simulink model "CG_Xilinxmodel"  (R2014a)
settings: Solver=ode45  StartTime=0.0  StopTime=0.12  RelTol=1e-3
undefined symbols (not defined in the file or in its folder): Down, Up
libraries: xbsIndex_r4 x102, powerlib x21
settings Model: Creator=Kiruba  LastModifiedBy=Acer
settings DebuggingCC: UnderspecifiedInitializationDetection=Classic

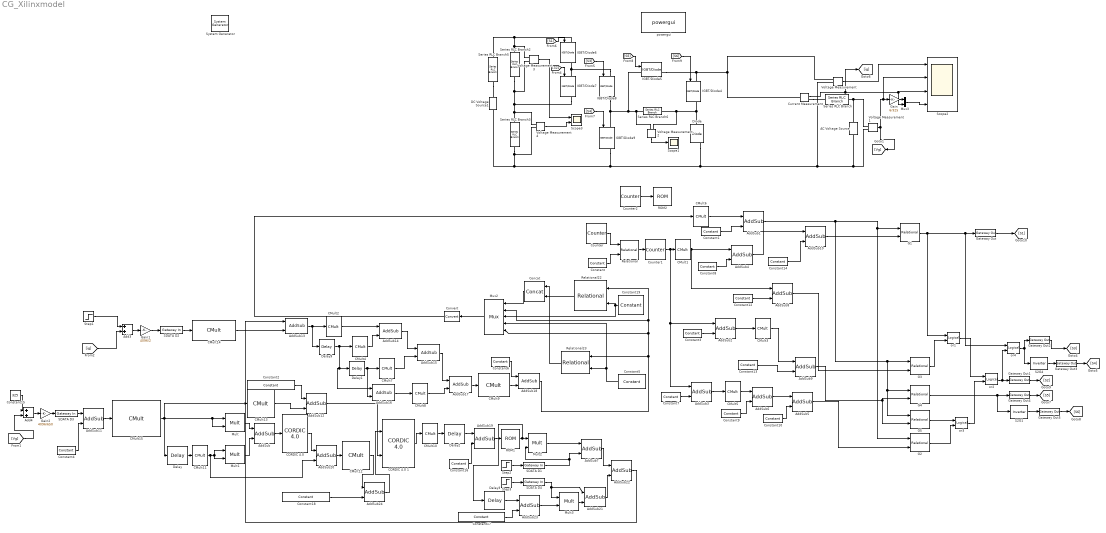
== system CG_Xilinxmodel ==
  " System Generator" : xbsIndex_r4/ System Generator  Tag=genX  xilinxfamily=spartan6  part=xc6slx45  speed=-3  package=csg324  synthesis_tool=XST  clock_wrapper=Clock Enables  directory=./netlist  proj_type=Project Navigator  Synth_file=XST Defaults  Impl_file=ISE Defaults  testbench=off  simulink_period=10e-9  sysclk_period=10  dcm_input_clock_period=10  incr_netlist=off  trim_vbits=Everywhere in SubSystem  dbl_ovrd=According to Block Masks  core_generation=According to Block Masks  run_coregen=off  deprecated_control=off  eval_field=0  block_type=sysgen
  AC Voltage Source : powerlib/Electrical Sources/AC Voltage Source  Amplitude=325  Phase=0  Frequency=50  SampleTime=0  Measurements=None
  Add3 : Sum
  Add4 : Sum
  AddSub : xbsIndex_r4/AddSub  mode=Addition  use_carryin=off  use_carryout=off  en=off  latency=0  precision=User Defined  arith_type=Unsigned  n_bits=18  bin_pt=0  quantization=Truncate  overflow=Wrap  dbl_ovrd=off  use_behavioral_HDL=off  hw_selection=Fabric  pipelined=off  block_type=addsub
  AddSub1 : xbsIndex_r4/AddSub  mode=Addition  use_carryin=off  use_carryout=off  en=off  latency=0  precision=Full  arith_type="Signed  (2's comp)"  n_bits=60  bin_pt=30  quantization=Truncate  overflow=Wrap  dbl_ovrd=off  use_behavioral_HDL=off  hw_selection=Fabric  pipelined=off  block_type=addsub
  AddSub10 : xbsIndex_r4/AddSub  mode=Addition  use_carryin=off  use_carryout=off  en=off  latency=0  precision=Full  arith_type="Signed  (2's comp)"  n_bits=60  bin_pt=30  quantization=Truncate  overflow=Wrap  dbl_ovrd=off  use_behavioral_HDL=off  hw_selection=Fabric  pipelined=off  block_type=addsub
  AddSub11 : xbsIndex_r4/AddSub  mode=Subtraction  use_carryin=off  use_carryout=off  en=off  latency=0  precision=Full  arith_type=Unsigned  n_bits=16  bin_pt=14  quantization=Truncate  overflow=Wrap  dbl_ovrd=off  use_behavioral_HDL=off  hw_selection=Fabric  pipelined=off  block_type=addsub
  AddSub12 : xbsIndex_r4/AddSub  mode=Addition  use_carryin=off  use_carryout=off  en=off  latency=0  precision=User Defined  arith_type="Signed  (2's comp)"  n_bits=32  bin_pt=30  quantization=Truncate  overflow=Wrap  dbl_ovrd=off  use_behavioral_HDL=off  hw_selection=Fabric  pipelined=off  block_type=addsub
  AddSub13 : xbsIndex_r4/AddSub  mode=Subtraction  use_carryin=off  use_carryout=off  en=off  latency=0  precision=Full  arith_type=Unsigned  n_bits=16  bin_pt=14  quantization=Truncate  overflow=Wrap  dbl_ovrd=off  use_behavioral_HDL=off  hw_selection=Fabric  pipelined=off  block_type=addsub
  AddSub{7,14..15,17..18,21..22} (7 alike) : xbsIndex_r4/AddSub  mode=Addition  use_carryin=off  use_carryout=off  en=off  latency=0  precision=Full  arith_type=Unsigned  n_bits=16  bin_pt=14  quantization=Truncate  overflow=Wrap  dbl_ovrd=off  use_behavioral_HDL=off  hw_selection=Fabric  pipelined=off  block_type=addsub
  AddSub16 : xbsIndex_r4/AddSub  mode=Subtraction  use_carryin=off  use_carryout=off  en=off  latency=1  precision=Full  arith_type=Unsigned  n_bits=16  bin_pt=14  quantization=Truncate  overflow=Wrap  dbl_ovrd=off  use_behavioral_HDL=off  hw_selection=Fabric  pipelined=off  block_type=addsub
  AddSub19 : xbsIndex_r4/AddSub  mode=Addition  use_carryin=off  use_carryout=off  en=off  latency=0  precision=User Defined  arith_type=Unsigned  n_bits=14  bin_pt=0  quantization=Truncate  overflow=Wrap  dbl_ovrd=off  use_behavioral_HDL=off  hw_selection=Fabric  pipelined=off  block_type=addsub
  AddSub2 : xbsIndex_r4/AddSub  mode=Subtraction  use_carryin=off  use_carryout=off  en=off  latency=0  precision=Full  arith_type=Unsigned  n_bits=13  bin_pt=0  quantization=Truncate  overflow=Wrap  dbl_ovrd=off  use_behavioral_HDL=off  hw_selection=Fabric  pipelined=off  block_type=addsub
  AddSub20 : xbsIndex_r4/AddSub  mode=Subtraction  use_carryin=off  use_carryout=off  en=off  latency=0  precision=Full  arith_type="Signed  (2's comp)"  n_bits=9  bin_pt=7  quantization=Truncate  overflow=Wrap  dbl_ovrd=off  use_behavioral_HDL=off  hw_selection=Fabric  pipelined=off  block_type=addsub
  AddSub23 : xbsIndex_r4/AddSub  mode=Addition  use_carryin=off  use_carryout=off  en=off  latency=0  precision=User Defined  arith_type="Signed  (2's comp)"  n_bits=32  bin_pt=30  quantization=Truncate  overflow=Wrap  dbl_ovrd=off  use_behavioral_HDL=off  hw_selection=Fabric  pipelined=off  block_type=addsub
  AddSub24 : xbsIndex_r4/AddSub  mode=Addition  use_carryin=off  use_carryout=off  en=off  latency=0  precision=User Defined  arith_type="Signed  (2's comp)"  n_bits=32  bin_pt=30  quantization=Truncate  overflow=Wrap  dbl_ovrd=off  use_behavioral_HDL=off  hw_selection=Fabric  pipelined=off  block_type=addsub
  AddSub3 : xbsIndex_r4/AddSub  mode=Subtraction  use_carryin=off  use_carryout=off  en=off  latency=0  precision=Full  arith_type=Unsigned  n_bits=13  bin_pt=0  quantization=Truncate  overflow=Wrap  dbl_ovrd=off  use_behavioral_HDL=off  hw_selection=Fabric  pipelined=off  block_type=addsub
  AddSub{4..5,8..9} (4 alike) : xbsIndex_r4/AddSub  mode=Addition  use_carryin=off  use_carryout=off  en=off  latency=0  precision=Full  arith_type=Unsigned  n_bits=13  bin_pt=0  quantization=Truncate  overflow=Wrap  dbl_ovrd=off  use_behavioral_HDL=off  hw_selection=Fabric  pipelined=off  block_type=addsub
  AddSub6 : xbsIndex_r4/AddSub  mode=Subtraction  use_carryin=off  use_carryout=off  en=off  latency=0  precision=Full  arith_type=Unsigned  n_bits=13  bin_pt=0  quantization=Truncate  overflow=Wrap  dbl_ovrd=off  use_behavioral_HDL=off  hw_selection=Fabric  pipelined=off  block_type=addsub
  CMult1 : xbsIndex_r4/CMult  const=0.5  gui_display_data_type=Fixed-point  const_n_bits=16  const_bin_pt=4  float_type=Single  exp_bits=8  fraction_bits=24  en=off  latency=0  precision=Full  arith_type="Signed  (2's comp)"  n_bits=16  bin_pt=14  quantization=Truncate  overflow=Wrap  dbl_ovrd=off  use_behavioral_HDL=off  mem_type=Distributed RAM  pipeline=off  block_type=cmult
      settings: block_version=12.1
  CMult10 : xbsIndex_r4/CMult  const=-250  gui_display_data_type=Fixed-point  const_n_bits=10  const_bin_pt=0  float_type=Single  exp_bits=8  fraction_bits=24  en=off  latency=0  precision=Full  arith_type="Signed  (2's comp)"  n_bits=16  bin_pt=14  quantization=Truncate  overflow=Wrap  dbl_ovrd=off  use_behavioral_HDL=off  mem_type=Distributed RAM  pipeline=off  block_type=cmult
      settings: block_version=12.1
  CMult11 : xbsIndex_r4/CMult  const=-1  gui_display_data_type=Fixed-point  const_n_bits=9  const_bin_pt=0  float_type=Single  exp_bits=8  fraction_bits=24  en=off  latency=0  precision=Full  arith_type="Signed  (2's comp)"  n_bits=16  bin_pt=14  quantization=Truncate  overflow=Wrap  dbl_ovrd=off  use_behavioral_HDL=off  mem_type=Distributed RAM  pipeline=off  block_type=cmult
      settings: block_version=12.1
  CMult12 : xbsIndex_r4/CMult  const=1/650  gui_display_data_type=Fixed-point  const_n_bits=32  const_bin_pt=30  float_type=Single  exp_bits=8  fraction_bits=24  en=off  latency=0  precision=User Defined  arith_type="Signed  (2's comp)"  n_bits=32  bin_pt=30  quantization=Truncate  overflow=Wrap  dbl_ovrd=off  use_behavioral_HDL=off  mem_type=Distributed RAM  pipeline=off  block_type=cmult
  CMult13 : xbsIndex_r4/CMult  const=1/650  gui_display_data_type=Fixed-point  const_n_bits=32  const_bin_pt=30  float_type=Single  exp_bits=8  fraction_bits=24  en=off  latency=0  precision=User Defined  arith_type="Signed  (2's comp)"  n_bits=9  bin_pt=7  quantization=Truncate  overflow=Wrap  dbl_ovrd=off  use_behavioral_HDL=off  mem_type=Distributed RAM  pipeline=off  block_type=cmult
  CMult14 : xbsIndex_r4/CMult  const=2/4096  gui_display_data_type=Fixed-point  const_n_bits=20  const_bin_pt=18  float_type=Single  exp_bits=8  fraction_bits=24  en=off  latency=0  precision=Full  arith_type="Signed  (2's comp)"  n_bits=16  bin_pt=14  quantization=Truncate  overflow=Wrap  dbl_ovrd=off  use_behavioral_HDL=off  mem_type=Distributed RAM  pipeline=off  block_type=cmult
      settings: block_version=12.1
  CMult15 : xbsIndex_r4/CMult  const=650/4101  gui_display_data_type=Fixed-point  const_n_bits=20  const_bin_pt=18  float_type=Single  exp_bits=8  fraction_bits=24  en=off  latency=0  precision=Full  arith_type="Signed  (2's comp)"  n_bits=16  bin_pt=14  quantization=Truncate  overflow=Wrap  dbl_ovrd=off  use_behavioral_HDL=off  mem_type=Distributed RAM  pipeline=off  block_type=cmult
      settings: block_version=12.1
  CMult2 : xbsIndex_r4/CMult  const=250.5  gui_display_data_type=Fixed-point  const_n_bits=10  const_bin_pt=2  float_type=Single  exp_bits=8  fraction_bits=24  en=off  latency=0  precision=Full  arith_type="Signed  (2's comp)"  n_bits=16  bin_pt=14  quantization=Truncate  overflow=Wrap  dbl_ovrd=off  use_behavioral_HDL=off  mem_type=Distributed RAM  pipeline=off  block_type=cmult
      settings: block_version=12.1
  CMult3 : xbsIndex_r4/CMult  const=0.5  gui_display_data_type=Fixed-point  const_n_bits=16  const_bin_pt=4  float_type=Single  exp_bits=8  fraction_bits=24  en=off  latency=0  precision=Full  arith_type="Signed  (2's comp)"  n_bits=16  bin_pt=14  quantization=Truncate  overflow=Wrap  dbl_ovrd=off  use_behavioral_HDL=off  mem_type=Distributed RAM  pipeline=off  block_type=cmult
      settings: block_version=12.1
  CMult4 : xbsIndex_r4/CMult  const=180.2  gui_display_data_type=Fixed-point  const_n_bits=10  const_bin_pt=2  float_type=Single  exp_bits=8  fraction_bits=24  en=off  latency=0  precision=Full  arith_type="Signed  (2's comp)"  n_bits=16  bin_pt=14  quantization=Truncate  overflow=Wrap  dbl_ovrd=off  use_behavioral_HDL=off  mem_type=Distributed RAM  pipeline=off  block_type=cmult
      settings: block_version=12.1
  CMult5 : xbsIndex_r4/CMult  const=0.5  gui_display_data_type=Fixed-point  const_n_bits=16  const_bin_pt=4  float_type=Single  exp_bits=8  fraction_bits=24  en=off  latency=0  precision=Full  arith_type="Signed  (2's comp)"  n_bits=16  bin_pt=14  quantization=Truncate  overflow=Wrap  dbl_ovrd=off  use_behavioral_HDL=off  mem_type=Distributed RAM  pipeline=off  block_type=cmult
      settings: block_version=12.1
  CMult6 : xbsIndex_r4/CMult  const=1250  gui_display_data_type=Fixed-point  const_n_bits=16  const_bin_pt=4  float_type=Single  exp_bits=8  fraction_bits=24  en=off  latency=0  precision=Full  arith_type="Signed  (2's comp)"  n_bits=16  bin_pt=14  quantization=Truncate  overflow=Wrap  dbl_ovrd=off  use_behavioral_HDL=off  mem_type=Distributed RAM  pipeline=off  block_type=cmult
      settings: block_version=12.1
  CMult7 : xbsIndex_r4/CMult  const=15.5  gui_display_data_type=Fixed-point  const_n_bits=10  const_bin_pt=2  float_type=Single  exp_bits=8  fraction_bits=24  en=off  latency=0  precision=Full  arith_type="Signed  (2's comp)"  n_bits=16  bin_pt=14  quantization=Truncate  overflow=Wrap  dbl_ovrd=off  use_behavioral_HDL=off  mem_type=Distributed RAM  pipeline=off  block_type=cmult
      settings: block_version=12.1
  CMult8 : xbsIndex_r4/CMult  const=2  gui_display_data_type=Fixed-point  const_n_bits=10  const_bin_pt=2  float_type=Single  exp_bits=8  fraction_bits=24  en=off  latency=0  precision=Full  arith_type="Signed  (2's comp)"  n_bits=16  bin_pt=14  quantization=Truncate  overflow=Wrap  dbl_ovrd=off  use_behavioral_HDL=off  mem_type=Distributed RAM  pipeline=off  block_type=cmult
      settings: block_version=12.1
  CMult9 : xbsIndex_r4/CMult  const=(1/400)  gui_display_data_type=Fixed-point  const_n_bits=14  const_bin_pt=12  float_type=Single  exp_bits=8  fraction_bits=24  en=off  latency=0  precision=Full  arith_type="Signed  (2's comp)"  n_bits=16  bin_pt=14  quantization=Truncate  overflow=Wrap  dbl_ovrd=off  use_behavioral_HDL=off  mem_type=Distributed RAM  pipeline=off  block_type=cmult
      settings: block_version=12.1
  "CORDIC 4.0 " : xbsIndex_r4/CORDIC 4.0   functional_selection=Square_Root  architectural_configuration=Parallel  pipelining_mode=Maximum  data_format=UnsignedInteger  phase_format=Radians  output_width=10  round_mode=Truncate  iterations=0  precision=0  coarse_rotation=off  compensation_scaling=No_Scale_Compensation  ce=off  sclr=off  nd=off  rdy=off  x_out=on  y_out=off  phase_output=off  register_inputs=true  register_outputs=true  ipcore_usecache=true  ipcore_useipmodelcache=true  ipcore_verbose=false  wrapper_available=true  ip_name=CORDIC  ip_version=4.0  dsptool_ready=true  port_translation_map={ 'ce' => 'en', 'sclr' => 'rst' }  structural_sim=false  block_type=cordic_v4_0
  CORDIC 4.0 1 : xbsIndex_r4/CORDIC 4.0   functional_selection=Arc_Tan  architectural_configuration=Parallel  pipelining_mode=No_Pipelining  data_format=SignedFraction  phase_format=Radians  output_width=40  round_mode=Truncate  iterations=0  precision=0  coarse_rotation=on  compensation_scaling=No_Scale_Compensation  ce=off  sclr=off  nd=off  rdy=off  x_out=off  y_out=off  phase_output=on  register_inputs=true  register_outputs=true  ipcore_usecache=true  ipcore_useipmodelcache=true  ipcore_verbose=false  wrapper_available=true  ip_name=CORDIC  ip_version=4.0  dsptool_ready=true  port_translation_map={ 'ce' => 'en', 'sclr' => 'rst' }  structural_sim=false  block_type=cordic_v4_0
  Concat : xbsIndex_r4/Concat  num_inputs=2  dbl_ovrd=off  block_type=concat
  Constant : xbsIndex_r4/Constant  const=1250  gui_display_data_type=Fixed-point  arith_type=Unsigned  n_bits=16  bin_pt=0  preci_type=Single  exp_width=8  frac_width=24  explicit_period=off  period=1  equ=P=C  opselect=C  inp2=PCIN>>17  opr=+  inp1=P  carry=CIN  dbl_ovrd=off  block_type=constant
  Constant1 : xbsIndex_r4/Constant  const=0  gui_display_data_type=Fixed-point  arith_type=Unsigned  n_bits=30  bin_pt=4  preci_type=Single  exp_width=8  frac_width=24  explicit_period=off  period=1  equ=P=C  opselect=C  inp2=PCIN>>17  opr=+  inp1=P  carry=CIN  dbl_ovrd=off  block_type=constant
      settings: block_version=12.1
  Constant{3,7,10,12..13} (5 alike) : xbsIndex_r4/Constant  const=1250  gui_display_data_type=Fixed-point  arith_type=Unsigned  n_bits=13  bin_pt=2  preci_type=Single  exp_width=8  frac_width=24  explicit_period=off  period=1  equ=P=C  opselect=C  inp2=PCIN>>17  opr=+  inp1=P  carry=CIN  dbl_ovrd=off  block_type=constant
      settings: block_version=12.1
  Constant14 : xbsIndex_r4/Constant  const=1250  gui_display_data_type=Fixed-point  arith_type=Unsigned  n_bits=30  bin_pt=4  preci_type=Single  exp_width=8  frac_width=24  explicit_period=off  period=1  equ=P=C  opselect=C  inp2=PCIN>>17  opr=+  inp1=P  carry=CIN  dbl_ovrd=off  block_type=constant
      settings: block_version=12.1
  Constant15 : Constant  Value=325
  Constant16 : xbsIndex_r4/Constant  const=393  gui_display_data_type=Fixed-point  arith_type=Unsigned  n_bits=10  bin_pt=0  preci_type=Single  exp_width=8  frac_width=24  explicit_period=off  period=1  equ=P=C  opselect=C  inp2=PCIN>>17  opr=+  inp1=P  carry=CIN  dbl_ovrd=off  block_type=constant
  Constant17 : xbsIndex_r4/Constant  const=0.06  gui_display_data_type=Fixed-point  arith_type=Signed (2's comp)  n_bits=32  bin_pt=30  preci_type=Single  exp_width=8  frac_width=24  explicit_period=off  period=1  equ=P=C  opselect=C  inp2=PCIN>>17  opr=+  inp1=P  carry=CIN  dbl_ovrd=off  block_type=constant
  Constant18 : xbsIndex_r4/Constant  const=0.00108  gui_display_data_type=Fixed-point  arith_type=Signed (2's comp)  n_bits=32  bin_pt=30  preci_type=Single  exp_width=8  frac_width=24  explicit_period=off  period=1  equ=P=C  opselect=C  inp2=PCIN>>17  opr=+  inp1=P  carry=CIN  dbl_ovrd=off  block_type=constant
  Constant19 : xbsIndex_r4/Constant  const=2  gui_display_data_type=Fixed-point  arith_type=Signed (2's comp)  n_bits=15  bin_pt=10  preci_type=Single  exp_width=8  frac_width=24  explicit_period=off  period=1  equ=P=C  opselect=C  inp2=PCIN>>17  opr=+  inp1=P  carry=CIN  dbl_ovrd=off  block_type=constant
  Constant2 : xbsIndex_r4/Constant  const=0.0062  gui_display_data_type=Fixed-point  arith_type=Signed (2's comp)  n_bits=32  bin_pt=30  preci_type=Single  exp_width=8  frac_width=24  explicit_period=off  period=1  equ=P=C  opselect=C  inp2=PCIN>>17  opr=+  inp1=P  carry=CIN  dbl_ovrd=off  block_type=constant
  Constant4 : xbsIndex_r4/Constant  const=4096/2  gui_display_data_type=Fixed-point  arith_type=Unsigned  n_bits=12  bin_pt=0  preci_type=Single  exp_width=8  frac_width=24  explicit_period=off  period=1  equ=P=C  opselect=C  inp2=PCIN>>17  opr=+  inp1=P  carry=CIN  dbl_ovrd=off  block_type=constant
      settings: block_version=12.1
  Constant5 : xbsIndex_r4/Constant  const=0.01  gui_display_data_type=Fixed-point  arith_type=Signed (2's comp)  n_bits=15  bin_pt=10  preci_type=Single  exp_width=8  frac_width=24  explicit_period=off  period=1  equ=P=C  opselect=C  inp2=PCIN>>17  opr=+  inp1=P  carry=CIN  dbl_ovrd=off  block_type=constant
  Constant6 : xbsIndex_r4/Constant  const=1  gui_display_data_type=Fixed-point  arith_type=Unsigned  n_bits=15  bin_pt=0  preci_type=Single  exp_width=8  frac_width=24  explicit_period=off  period=1  equ=P=C  opselect=C  inp2=PCIN>>17  opr=+  inp1=P  carry=CIN  dbl_ovrd=off  block_type=constant
  Constant8 : xbsIndex_r4/Constant  const=625  gui_display_data_type=Fixed-point  arith_type=Unsigned  n_bits=13  bin_pt=2  preci_type=Single  exp_width=8  frac_width=24  explicit_period=off  period=1  equ=P=C  opselect=C  inp2=PCIN>>17  opr=+  inp1=P  carry=CIN  dbl_ovrd=off  block_type=constant
      settings: block_version=12.1
  Constant9 : xbsIndex_r4/Constant  const=625  gui_display_data_type=Fixed-point  arith_type=Unsigned  n_bits=13  bin_pt=2  preci_type=Single  exp_width=8  frac_width=24  explicit_period=off  period=1  equ=P=C  opselect=C  inp2=PCIN>>17  opr=+  inp1=P  carry=CIN  dbl_ovrd=off  block_type=constant
      settings: block_version=12.1
  Convert : xbsIndex_r4/Convert  gui_display_data_type=Fixed-point  arith_type=Unsigned  n_bits=16  bin_pt=14  float_type=Single  exp_bits=8  fraction_bits=24  quantization=Truncate  overflow=Wrap  en=off  latency=0  dbl_ovrd=off  pipeline=off  block_type=convert
  Counter : xbsIndex_r4/Counter  cnt_type=Count Limited  cnt_to=2500  operation=Up  start_count=1  cnt_by_val=1  arith_type=Unsigned  n_bits=13  bin_pt=0  load_pin=off  rst=off  en=off  explicit_period=on  period=8e-8  dbl_ovrd=off  use_behavioral_HDL=off  implementation=Fabric  block_type=counter
  Counter1 : xbsIndex_r4/Counter  cnt_type=Count Limited  cnt_to=2500  operation=Up/Down  start_count=1  cnt_by_val=1  arith_type=Unsigned  n_bits=13  bin_pt=0  load_pin=off  rst=off  en=off  explicit_period=on  period=8e-8  dbl_ovrd=off  use_behavioral_HDL=off  implementation=Fabric  block_type=counter
  Counter2 : xbsIndex_r4/Counter  cnt_type=Count Limited  cnt_to=1000  operation=Up  start_count=1  cnt_by_val=1  arith_type=Unsigned  n_bits=14  bin_pt=0  load_pin=off  rst=off  en=off  explicit_period=on  period=20e-6  dbl_ovrd=off  use_behavioral_HDL=off  implementation=Fabric  block_type=counter
      settings: block_version=12.1
  Current Measurement : powerlib/Measurements/Current Measurement  PhasorSimulation=off  OutputType=Complex  PSBequivalent=0
  DC Voltage Source1 : powerlib/Electrical Sources/DC Voltage Source  Amplitude=400  Measurements=None
  Delay : xbsIndex_r4/Delay  rst=off  infoeditControl=Selection of Reset will increase slice count due to use of real FFs and instead of SRLs  en=off  latency=560  dbl_ovrd=off  reg_retiming=off  block_type=delay
  Delay1 : xbsIndex_r4/Delay  rst=off  infoeditControl=Selection of Reset will increase slice count due to use of real FFs and instead of SRLs  en=off  latency=1  dbl_ovrd=off  reg_retiming=off  block_type=delay
  Delay2 : xbsIndex_r4/Delay  rst=off  infoeditControl=Selection of Reset will increase slice count due to use of real FFs and instead of SRLs  en=off  latency=560  dbl_ovrd=off  reg_retiming=off  block_type=delay
  Delay3 : xbsIndex_r4/Delay  rst=off  infoeditControl=Selection of Reset will increase slice count due to use of real FFs and instead of SRLs  en=off  latency=560  dbl_ovrd=off  reg_retiming=off  block_type=delay
  Delay9 : xbsIndex_r4/Delay  rst=off  infoeditControl=Selection of Reset will increase slice count due to use of real FFs and instead of SRLs  en=off  latency=1  dbl_ovrd=off  reg_retiming=off  block_type=delay
  Diode : powerlib/Power Electronics/Diode  Ron=0.001  Lon=0  Vf=0.8  IC=0  UseSnubber=off  Rs=500  Cs=250e-9  Measurements=on
  G1 : xbsIndex_r4/Relational  mode=a>=b  en=off  latency=1  dbl_ovrd=off  block_type=relational
      settings: block_version=12.1
  G2 : xbsIndex_r4/Relational  mode=a<=b  en=off  latency=1  dbl_ovrd=off  block_type=relational
      settings: block_version=12.1
  G3 : xbsIndex_r4/Relational  mode=a>=b  en=off  latency=1  dbl_ovrd=off  block_type=relational
      settings: block_version=12.1
  G4 : xbsIndex_r4/Relational  mode=a>=b  en=off  latency=1  dbl_ovrd=off  block_type=relational
      settings: block_version=12.1
  G5 : xbsIndex_r4/Relational  mode=a<=b  en=off  latency=1  dbl_ovrd=off  block_type=relational
      settings: block_version=12.1
  Gain : Gain  Gain=6/325
  Gain1 : Gain  Gain=4096/2
  Gain2 : Gain  Gain=4096/650
  Gateway Out : xbsIndex_r4/Gateway Out  inherit_from_input=off  hdl_port=on  timing_constraint=None  locs_specified=on  LOCs={'U16'}  UseAsDAC=off  DACChannel='1'  block_type=gatewayout
  Gateway Out1 : xbsIndex_r4/Gateway Out  inherit_from_input=off  hdl_port=on  timing_constraint=None  locs_specified=on  LOCs={'U15'}  UseAsDAC=off  DACChannel='1'  block_type=gatewayout
  Gateway Out2 : xbsIndex_r4/Gateway Out  inherit_from_input=off  hdl_port=on  timing_constraint=None  locs_specified=on  LOCs={'U13'}  UseAsDAC=off  DACChannel='1'  block_type=gatewayout
  Gateway Out3 : xbsIndex_r4/Gateway Out  inherit_from_input=off  hdl_port=on  timing_constraint=None  locs_specified=on  LOCs={'M11'}  UseAsDAC=off  DACChannel='1'  block_type=gatewayout
  Gateway Out4 : xbsIndex_r4/Gateway Out  inherit_from_input=off  hdl_port=on  timing_constraint=None  locs_specified=on  LOCs={'R11'}  UseAsDAC=off  DACChannel='1'  block_type=gatewayout
  Gateway Out5 : xbsIndex_r4/Gateway Out  inherit_from_input=off  hdl_port=on  timing_constraint=None  locs_specified=on  LOCs={'T12'}  UseAsDAC=off  DACChannel='1'  block_type=gatewayout
  IGBT/Diode{4..9} (6 alike) : powerlib/Power Electronics/IGBT//Diode  Ron=1e-3  Rs=1e5  Cs=inf  Measurements=on
  Mult{,1..3} (4 alike) : xbsIndex_r4/Mult  precision=Full  arith_type="Signed  (2's comp)"  n_bits=16  bin_pt=14  quantization=Truncate  overflow=Wrap  en=off  latency=0  dbl_ovrd=off  use_behavioral_HDL=off  opt=Speed  use_embedded=on  optimum_pipeline=off  pipeline=on  use_rpm=on  placement_style=Triangular  block_type=mult
  Mux2 : xbsIndex_r4/Mux  inputs=4  en=off  latency=0  precision=Full  arith_type=Unsigned  n_bits=16  bin_pt=2  quantization=Truncate  overflow=Wrap  dbl_ovrd=off  block_type=mux
  Mux3 : Mux  Inputs=2
  ROM1 : xbsIndex_r4/ROM  depth=16384  initVector=cos( 2*pi*(0:785)/786)  distributed_mem=Block RAM  rst=off  init_reg=0  en=off  latency=1  gui_display_data_type=Fixed-point  arith_type="Signed  (2's comp)"  n_bits=16  bin_pt=14  preci_type=Single  exp_width=8  frac_width=24  dbl_ovrd=off  optimize=Area  use_rpm=on  block_type=sprom
      settings: block_version=8.2.02
  ROM2 : xbsIndex_r4/ROM  depth=16384  initVector=sin( 2*pi*(0:999)/1000)  distributed_mem=Block RAM  rst=off  init_reg=0  en=off  latency=1  gui_display_data_type=Fixed-point  arith_type="Signed  (2's comp)"  n_bits=16  bin_pt=14  preci_type=Single  exp_width=8  frac_width=24  dbl_ovrd=off  optimize=Area  use_rpm=on  block_type=sprom
      settings: block_version=8.2.02
  Relational : xbsIndex_r4/Relational  mode=a<=b  en=off  latency=0  dbl_ovrd=off  block_type=relational
  Relational22 : xbsIndex_r4/Relational  mode=a>b  en=off  latency=0  dbl_ovrd=off  block_type=relational
  Relational23 : xbsIndex_r4/Relational  mode=a<b  en=off  latency=0  dbl_ovrd=off  block_type=relational
  S2G1 : xbsIndex_r4/Inverter  en=off  latency=0  dbl_ovrd=off  block_type=inv
      settings: block_version=12.1
  S2G4 : xbsIndex_r4/Inverter  en=off  latency=0  dbl_ovrd=off  block_type=inv
      settings: block_version=12.1
  SDATA D1 : xbsIndex_r4/Gateway In  gui_display_data_type=Fixed-point  arith_type=Unsigned  n_bits=16  bin_pt=4  preci_type=Single  exp_width=8  frac_width=24  quantization="Round  (unbiased: +/- Inf)"  overflow=Saturate  period=2*44e-7  dbl_ovrd=off  timing_constraint=Data Rate  locs_specified=off  LOCs={'R3'}  UseAsADC=off  ADCChannel='1'  inherit_from_input=off  hdl_port=on  block_type=gatewayin
  SDATA D2 : xbsIndex_r4/Gateway In  gui_display_data_type=Fixed-point  arith_type=Unsigned  n_bits=32  bin_pt=4  preci_type=Single  exp_width=8  frac_width=24  quantization="Round  (unbiased: +/- Inf)"  overflow=Saturate  period=2*44e-7  dbl_ovrd=off  timing_constraint=Data Rate  locs_specified=off  LOCs={'R3'}  UseAsADC=off  ADCChannel='1'  inherit_from_input=off  hdl_port=on  block_type=gatewayin
  SDATA D3 : xbsIndex_r4/Gateway In  gui_display_data_type=Fixed-point  arith_type=Unsigned  n_bits=16  bin_pt=0  preci_type=Single  exp_width=8  frac_width=24  quantization="Round  (unbiased: +/- Inf)"  overflow=Saturate  period=2*44e-7  dbl_ovrd=off  timing_constraint=Data Rate  locs_specified=off  LOCs={'R3'}  UseAsADC=off  ADCChannel='1'  inherit_from_input=off  hdl_port=on  block_type=gatewayin
  SDATA D4 : xbsIndex_r4/Gateway In  gui_display_data_type=Fixed-point  arith_type=Unsigned  n_bits=16  bin_pt=4  preci_type=Single  exp_width=8  frac_width=24  quantization="Round  (unbiased: +/- Inf)"  overflow=Saturate  period=2*44e-7  dbl_ovrd=off  timing_constraint=Data Rate  locs_specified=off  LOCs={'R3'}  UseAsADC=off  ADCChannel='1'  inherit_from_input=off  hdl_port=on  block_type=gatewayin
  Scope1 : Scope
      settings: TimeRange=0.1  YMin=94.2  YMax=95.9  SaveName=ScopeData2
  Scope2 : Scope  NumInputPorts=4
      settings: TimeRange=0.04  YMin=-25~45~0.2~0.2  YMax=200~65~0.85~1.2  SaveName=ScopeData4
  Scope3 : Scope  NumInputPorts=2
      settings: TimeRange=0.1  YMin=235.275~164.225  YMax=235.575~164.55  SaveName=ScopeData3
  Series RLC Branch : powerlib/Elements/Series RLC Branch  LConnTagsString=__new0  RConnTagsString=__new0  BranchType=RL  Resistance=0.02  Inductance=10e-3  SetiL0=off  InitialCurrent=0  Capacitance=1e-6  Setx0=off  InitialVoltage=0  Measurements=None
  Series RLC Branch2 : powerlib/Elements/Series RLC Branch  LConnTagsString=__new0  RConnTagsString=__new0  BranchType=RC  Resistance=0.01  Inductance=6e-3  SetiL0=off  InitialCurrent=0  Capacitance=2000e-6  Setx0=off  InitialVoltage=0  Measurements=None
  Series RLC Branch3 : powerlib/Elements/Series RLC Branch  LConnTagsString=__new0  RConnTagsString=__new0  BranchType=RC  Resistance=0.01  Inductance=6e-3  SetiL0=off  InitialCurrent=0  Capacitance=2000e-6  Setx0=off  InitialVoltage=0  Measurements=None
  Series RLC Branch5 : powerlib/Elements/Series RLC Branch  LConnTagsString=__new0  RConnTagsString=__new0  BranchType=R  Resistance=0.01  Inductance=6e-3  SetiL0=off  InitialCurrent=0  Capacitance=1000e-6  Setx0=off  InitialVoltage=0  Measurements=None
  Series RLC Branch6 : powerlib/Elements/Series RLC Branch  LConnTagsString=__new0  RConnTagsString=__new0  BranchType=C  Resistance=0.00002  Inductance=6e-3  SetiL0=off  InitialCurrent=0  Capacitance=2000e-6  Setx0=off  InitialVoltage=100  Measurements=None
  Step1 : Step  Time=0.06  Before=5  After=5  SampleTime=0
  Step2 : Step  Time=0.06  Before=5  After=0  SampleTime=0
  Step3 : Step  Time=0.06  After=5  SampleTime=0
  Voltage Measurement{,1..4} (5 alike) : powerlib/Measurements/Voltage Measurement  PhasorSimulation=off  OutputType=Complex  PSBequivalent=0
  or1 : xbsIndex_r4/Logical  logical_function=XOR  inputs=2  en=off  latency=0  precision=Full  arith_type=Unsigned  n_bits=16  bin_pt=0  align_bp=on  dbl_ovrd=off  block_type=logical
      settings: block_version=12.1
  or2 : xbsIndex_r4/Logical  logical_function=OR  inputs=2  en=off  latency=0  precision=Full  arith_type=Unsigned  n_bits=16  bin_pt=0  align_bp=on  dbl_ovrd=off  block_type=logical
      settings: block_version=12.1
  or3 : xbsIndex_r4/Logical  logical_function=XOR  inputs=2  en=off  latency=0  precision=Full  arith_type=Unsigned  n_bits=16  bin_pt=0  align_bp=on  dbl_ovrd=off  block_type=logical
      settings: block_version=12.1
  or4 : xbsIndex_r4/Logical  logical_function=OR  inputs=2  en=off  latency=0  precision=Full  arith_type=Unsigned  n_bits=16  bin_pt=0  align_bp=on  dbl_ovrd=off  block_type=logical
      settings: block_version=12.1
  powergui : powerlib/powergui  Priority=1  SimulationMode=Discrete  SolverType=Tustin  SampleTime=1e-6  frequency=60  SPID=off  DisableSnubberDevices=off  DisableRonSwitches=off  DisableVfSwitches=off  SwTol=0  Interpol=off  DisplayEquations=off  Ts=0  methode=off  frequencyindice=0  Pbase=100e6  ErrMax=1e-4  Iterations=50  UnitsV=kV  UnitsW=MW  FunctionMessages=off  echomessages=off  HookPort=off  EnableUseOfTLC=off  x0status=blocks  RestoreLinks=warning  ResistiveCurrentMeasurement=off  Frange=[0:2:500]  Ylog=off  Xlog=on  ShowGrid=off  save=off  variable=ZData  structure=ScopeData  ZoomFFT=on  StartTime=0.02  cycles=2  DisplayStyle=1  fundamental=50  FreqAxis=off  MaxFrequency=10000  frequencyindicesteady=1  RmsSteady=1  display=off
  wires:
  Constant/1 -> Relational/2
  Relational/1 -> Counter1/1
  Counter/1 -> Relational/1
  Constant7/1 -> AddSub3/2
  CMult5/1 -> AddSub6/1
  Constant9/1 -> AddSub6/2
  AddSub6/1 -> AddSub5/1
  Constant10/1 -> AddSub5/2
  AddSub2/1 -> CMult3/1
  Constant3/1 -> AddSub2/2
  Constant13/1 -> AddSub9/2
  Constant12/1 -> AddSub8/2
  Counter1/1 -> CMult1/1, AddSub3/1, AddSub2/1
  AddSub4/1 -> AddSub10/1
  CMult1/1 -> AddSub4/1, AddSub8/1
  Constant8/1 -> AddSub4/2
  Constant14/1 -> AddSub10/2
  AddSub10/1 -> G1/2
  AddSub8/1 -> G3/2
  AddSub9/1 -> G4/2, G5/2
  AddSub5/1 -> G2/2
  AddSub3/1 -> CMult5/1
  CMult3/1 -> AddSub9/1
  G1/1 -> Gateway Out/1, or4/1, or1/1
  G3/1 -> or1/2
  G5/1 -> or3/1
  G2/1 -> or3/2
  or1/1 -> or2/1
  or3/1 -> or2/2
  or2/1 -> Gateway Out1/1, or4/2
  or4/1 -> Gateway Out2/1, S2G4/1
  S2G4/1 -> Gateway Out3/1
  G4/1 -> S2G1/1, Gateway Out4/1
  S2G1/1 -> Gateway Out5/1
  AddSub1/1 -> G1/1, G2/1, G3/1, G5/1, G4/1
  Counter2/1 -> ROM2/1
  Constant1/1 -> AddSub1/2
  CMult6/1 -> AddSub1/1
  Voltage Measurement/1 -> Scope2/1
  Voltage Measurement1/1 -> [Vg], Gain/1, Scope2/2
  Current Measurement/1 -> Mux3/2, Scope2/3, [ig]
  [S2] -> IGBT/Diode7/1
  [S1] -> IGBT/Diode6/1
  [S3] -> IGBT/Diode8/1
  [S4] -> IGBT/Diode9/1
  [S5] -> IGBT/Diode5/1
  [S6] -> IGBT/Diode4/1
  Voltage Measurement2/1 -> Scope1/1
  Voltage Measurement3/1 -> Scope3/1
  Voltage Measurement4/1 -> Scope3/2
  Mux3/1 -> Scope2/4
  Gain/1 -> Mux3/1
  Mux2/1 -> Convert/1
  AddSub13/1 -> Delay9/1, CMult2/1
  Delay9/1 -> Delay1/1, AddSub16/1, CMult4/1
  Delay1/1 -> CMult7/1, AddSub16/2
  CMult2/1 -> AddSub14/1
  CMult4/1 -> AddSub14/2
  AddSub14/1 -> AddSub15/1
  CMult7/1 -> AddSub15/2
  AddSub16/1 -> CMult8/1
  CMult8/1 -> AddSub17/2
  AddSub15/1 -> AddSub17/1
  AddSub17/1 -> CMult9/1
  [ig] -> Add3/2
  Step1/1 -> Add3/1
  Add3/1 -> Gain1/1
  SDATA D2/1 -> CMult14/1
  CMult9/1 -> AddSub18/2
  Constant6/1 -> AddSub18/1
  Concat/1 -> Mux2/1
  Relational23/1 -> Concat/1
  Relational22/1 -> Concat/2
  Constant19/1 -> Mux2/3, Relational22/2
  AddSub18/1 -> Relational23/1, Mux2/5, Relational22/1, Mux2/2
  Constant5/1 -> Relational23/2, Mux2/4
  [Vg] -> Add4/2
  Add4/1 -> Gain2/1
  AddSub11/1 -> CMult15/1
  Constant4/1 -> AddSub11/2
  CMult11/1 -> Mult1/2, Mult1/1, AddSub20/2
  Mult/1 -> AddSub/1
  Mult1/1 -> AddSub/2
  AddSub/1 -> "CORDIC 4.0 "/1
  "CORDIC 4.0 "/1 -> AddSub20/1
  AddSub20/1 -> CMult12/1
  Delay/1 -> CMult11/1
  CORDIC 4.0 1/1 -> CMult10/1
  CMult10/1 -> Delay2/1
  Constant16/1 -> AddSub19/2
  ROM1/1 -> Delay3/1, Mult2/1
  Mult2/1 -> AddSub7/1
  AddSub19/1 -> ROM1/1
  Delay2/1 -> AddSub19/1
  AddSub12/1 -> CORDIC 4.0 1/2
  CMult13/1 -> AddSub12/2
  Constant2/1 -> AddSub12/1
  Step2/1 -> SDATA D1/1
  Convert/1 -> CMult6/1
  Mult3/1 -> AddSub21/2
  AddSub21/1 -> AddSub22/2
  AddSub7/1 -> AddSub22/1
  AddSub22/1 -> AddSub13/1
  Step3/1 -> SDATA D4/1
  Delay3/1 -> AddSub23/1
  Constant17/1 -> AddSub23/2
  AddSub23/1 -> Mult3/2
  Gain1/1 -> SDATA D2/1
  CMult14/1 -> AddSub13/2
  Constant15/1 -> Add4/1
  Gain2/1 -> SDATA D3/1
  SDATA D3/1 -> AddSub11/1
  CMult15/1 -> Delay/1, Mult/1, Mult/2, CMult13/1
  Constant18/1 -> AddSub24/2
  CMult12/1 -> AddSub24/1
  AddSub24/1 -> CORDIC 4.0 1/1
  SDATA D1/1 -> AddSub7/2, Mult2/2
  SDATA D4/1 -> AddSub21/1, Mult3/1
  Gateway Out/1 -> [S1]
  Gateway Out1/1 -> [S2]
  Gateway Out2/1 -> [S3]
  Gateway Out3/1 -> [S4]
  Gateway Out4/1 -> [S5]
  Gateway Out5/1 -> [S6]
  connections:
  Diode/RConn1 -- IGBT/Diode9/RConn1 -- Series RLC Branch3/RConn1 -- Voltage Measurement4/LConn2 -- DC Voltage Source1/LConn1 -- Voltage Measurement/LConn2 -- Voltage Measurement1/LConn2 -- AC Voltage Source/LConn1
  Voltage Measurement1/LConn1 -- Series RLC Branch/RConn1 -- AC Voltage Source/RConn1
  Voltage Measurement3/LConn2 -- Series RLC Branch2/RConn1 -- Series RLC Branch3/LConn1 -- Voltage Measurement4/LConn1 -- IGBT/Diode7/RConn1
  Series RLC Branch5/LConn1 -- IGBT/Diode6/LConn1 -- Series RLC Branch2/LConn1 -- Voltage Measurement3/LConn1
  IGBT/Diode8/LConn1 -- IGBT/Diode6/RConn1 -- IGBT/Diode7/LConn1
  Voltage Measurement2/LConn1 -- Series RLC Branch6/LConn1 -- IGBT/Diode5/LConn1 -- IGBT/Diode8/RConn1 -- IGBT/Diode9/LConn1
  Voltage Measurement2/LConn2 -- Series RLC Branch6/RConn1 -- Diode/LConn1 -- IGBT/Diode4/RConn1
  Current Measurement/RConn1 -- Series RLC Branch/LConn1
  Series RLC Branch5/RConn1 -- DC Voltage Source1/RConn1
  Voltage Measurement/LConn1 -- Current Measurement/LConn1 -- IGBT/Diode4/LConn1 -- IGBT/Diode5/RConn1
